simulink model "homing"  (R2017a)
settings: Solver=FixedStepAuto  StartTime=0.0  StopTime=inf  FixedStep=1e-3  RelTol=1e-3  EnableMultiTasking=on
libraries: xpcnilib x12, simulink x4
settings Model: SimulationMode=external  Creator=Davide  LastModifiedBy=stefa
settings SolverCC: EnableConcurrentExecution=on  ConcurrentTasks=on  AutoInsertRateTranBlk=on
settings DataIOCC: SaveFormat=StructureWithTime
settings OptimizationCC: BlockReduction=off  OptimizeBlockIOStorage=off  BufferReuse=off  GlobalBufferReuse=off  ExpressionFolding=off  LocalBlockOutputs=off
settings HardwareCC: ProdBitPerPointer=32  ProdBitPerSizeT=32  ProdBitPerPtrDiffT=32  ProdLargestAtomicFloat=None  ProdWordSize=32  ProdLongLongMode=on  ProdHWDeviceType=Generic->32-bit x86 compatible
settings RTWCC: SystemTargetFile=slrt.tlc  TemplateMakefile=slrt_default_tmf  Description=Simulink Real-Time  RTWCompilerOptimization=on
settings SimulinkRealTimeCC: xPCConcurrentTasks=on

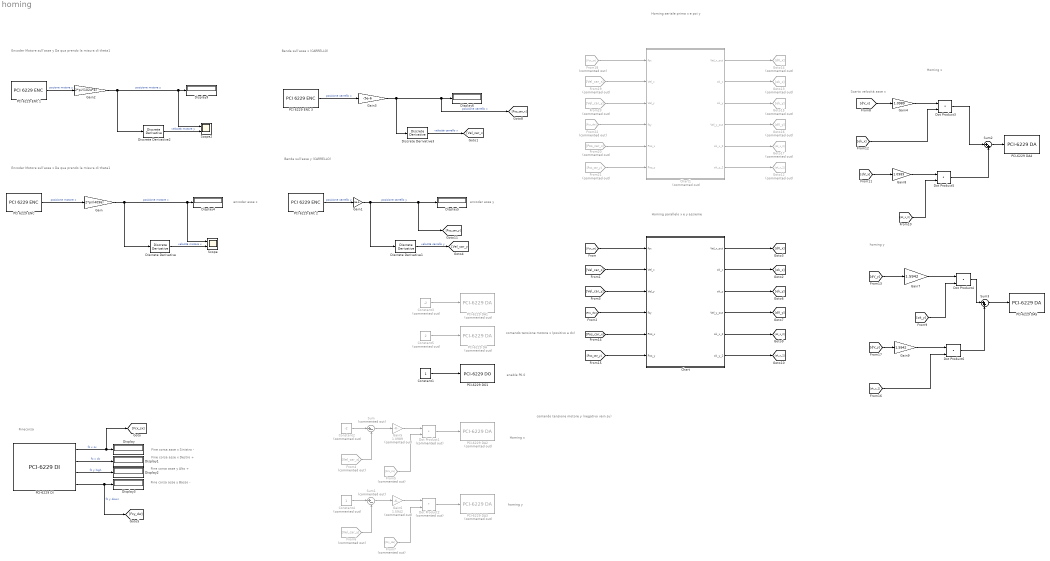
== system homing ==
  note: Homing seriale
      | prima x e poi y
  note: Scarto velocità asse x
  note: Encoder Motore sull'asse x
      | Da qua prendo la misura di theta1
  note: Fine corsa asse x Sinistro -
  note: homing y
  note: Homing x
  note: enable P0.0
  note: comando tensione motore x (positivo a dx)
  note: comando tensione motore y (negativo vain su)
  note: Finecorsa
  note: encoder asse y
  note: encoder asse x
  note: Fine corsa asse x Destro +
  note: Fine corsa asse y Alto +
  note: Fine corsa asse y Basso -
  note: Encoder Motore sull'asse y
      | Da qua prendo la misura di theta1
  note: Banda sull'asse x (CARRELLO)
  note: Banda sull'asse y (CARRELLO)
  note: Homing x
  note: homing y
  note: Homing parallelo
      | x e y assieme
  Chart : Stateflow chart  TreatAsAtomicUnit=on
  Chart1 : Stateflow chart  Commented=on  TreatAsAtomicUnit=on
  Constant1 : Constant
  Constant2 : Constant  Commented=on  Value=-2
  Constant3 : Constant  Commented=on  Value=-2
  Constant4 : Constant  Commented=on
  Constant5 : Constant  Commented=on  Value=2
  Discrete Derivative{,1..3} (4 alike) : simulink/Discrete/Discrete Derivative  gainval=1.0  ICPrevScaledInput=0.0  OutMin=[]  OutMax=[]  OutDataType=fixdt(1, 16)  OutScaling=2^-10  DoSatur=off
  Display{,1..6,9} (8 alike) : Display
  Dot Product1 : DotProduct  Commented=on  InputSameDT=on  OutDataTypeStr=Inherit: Inherit via internal rule
  Dot Product2 : DotProduct  Commented=on  InputSameDT=on  OutDataTypeStr=Inherit: Inherit via internal rule
  Dot Product{3..6} (4 alike) : DotProduct  InputSameDT=on  OutDataTypeStr=Inherit: Inherit via internal rule
  From18 : From  Commented=on  GotoTag=Fcx_sx
  From19 : From  Commented=on  GotoTag=Vel_car_x
  From20 : From  Commented=on  GotoTag=Pos_car_x
  From21 : From  Commented=on  GotoTag=Pos_car_y
  From22 : From  Commented=on  GotoTag=Fcy_dw
  From23 : From  Commented=on  GotoTag=Vel_car_y
  From4 : From  Commented=on  GotoTag=Vel_car_x
  From5 : From  Commented=on  GotoTag=Fcx_sx
  From6 : From  Commented=on  GotoTag=Vel_car_y
  From7 : From  Commented=on  GotoTag=Fcy_dw
  Gain : Gain  Gain=2*pi/(4096)
  Gain1 : Gain  Gain=-5e-6
  Gain2 : Gain  Gain=2*pi/(1024*4)
  Gain3 : Gain  Gain=-5e-6
  Gain4 : Gain  Gain=1.0989
  Gain5 : Gain  Commented=on  Gain=1.0989
  Gain6 : Gain  Commented=on  Gain=1.5942
  Gain7 : Gain  Gain=1.5942
  Gain8 : Gain  Gain=1.0989
  Gain9 : Gain  Gain=1.5942
  Goto12 : Goto  Commented=on  GotoTag=ok_y_2
  Goto13 : Goto  Commented=on  GotoTag=ok_x
  Goto14 : Goto  Commented=on  GotoTag=dV_x
  Goto15 : Goto  Commented=on  GotoTag=ok_y
  Goto16 : Goto  Commented=on  GotoTag=dV_y
  Goto17 : Goto  Commented=on  GotoTag=ok_x_2
  "PCI 6229 ENC " : xpcnilib/Incremental Encoder/PCI 6229 ENC   channel=0  countMode=Quadrature Mode x4  initCount=0  reload=on  indexPhase=A low B low  filter=None  sampleTime=0.001  slot=[4 12]
      settings: SourceProductName=Simulink Real-Time  SourceProductBaseCode=XP
  PCI 6229 ENC 1 : xpcnilib/Incremental Encoder/PCI 6229 ENC   channel=1  countMode=Quadrature Mode x4  initCount=0  reload=on  indexPhase=A low B low  filter=None  sampleTime=0.001  slot=[4 12]
      settings: SourceProductName=Simulink Real-Time  SourceProductBaseCode=XP
  PCI 6229 ENC 2 : xpcnilib/Incremental Encoder/PCI 6229 ENC   channel=0  countMode=Quadrature Mode x4  initCount=0  reload=on  indexPhase=A low B low  filter=None  sampleTime=0.001  slot=[4 15]
      settings: SourceProductName=Simulink Real-Time  SourceProductBaseCode=XP
  PCI 6229 ENC 3 : xpcnilib/Incremental Encoder/PCI 6229 ENC   channel=1  countMode=Quadrature Mode x4  initCount=0  reload=on  indexPhase=A low B low  filter=None  sampleTime=0.001  slot=[4 15]
      settings: SourceProductName=Simulink Real-Time  SourceProductBaseCode=XP
  PCI-6229 DA : xpcnilib/D//A/M Series/PCI-6229 DA  Commented=on  channel=[1]  reset=[1]  initValue=[0]  sampletime=0.001  slot=[4 12]
      settings: SourceProductName=Simulink Real-Time  SourceProductBaseCode=XP
  PCI-6229 DA1 : xpcnilib/D//A/M Series/PCI-6229 DA  Commented=on  channel=[1]  reset=[1]  initValue=[0]  sampletime=0.001  slot=[4 15]
      settings: SourceProductName=Simulink Real-Time  SourceProductBaseCode=XP
  PCI-6229 DA2 : xpcnilib/D//A/M Series/PCI-6229 DA  Commented=on  channel=[1]  reset=[1]  initValue=[0]  sampletime=0.001  slot=[4 12]
      settings: SourceProductName=Simulink Real-Time  SourceProductBaseCode=XP
  PCI-6229 DA3 : xpcnilib/D//A/M Series/PCI-6229 DA  Commented=on  channel=[1]  reset=[1]  initValue=[0]  sampletime=0.001  slot=[4 15]
      settings: SourceProductName=Simulink Real-Time  SourceProductBaseCode=XP
  PCI-6229 DA4 : xpcnilib/D//A/M Series/PCI-6229 DA  channel=[1]  reset=[1]  initValue=[0]  sampletime=0.001  slot=[4 12]
      settings: SourceProductName=Simulink Real-Time  SourceProductBaseCode=XP
  PCI-6229 DA5 : xpcnilib/D//A/M Series/PCI-6229 DA  channel=[1]  reset=[1]  initValue=[0]  sampletime=0.001  slot=[4 15]
      settings: SourceProductName=Simulink Real-Time  SourceProductBaseCode=XP
  PCI-6229 DI : xpcnilib/Digital Input/M Series/PCI-6229 DI  channel=[4 5 6 7]  sampletime=0.001  slot=[4 12]
      settings: SourceProductName=Simulink Real-Time  SourceProductBaseCode=XP
  PCI-6229 DO1 : xpcnilib/Digital Output/M Series/PCI-6229 DO  channel=[1]  reset=[1]  initValue=[0]  sampletime=0.001  slot=[4 12]
      settings: SourceProductName=Simulink Real-Time  SourceProductBaseCode=XP
  Scope : Scope  NumInputPorts=2
  Scope2 : Scope  NumInputPorts=2
  Sum : Sum  Commented=on  Inputs=|+-
  Sum1 : Sum  Commented=on  Inputs=|+-
  Sum2 : Sum  Inputs=|++
  Sum3 : Sum  Inputs=|++
  wires:
  PCI-6229 DI/1 -> [Fcx_sx], Display/1  "fc x sx"
  PCI-6229 DI/2 -> Display1/1  "fc x dx"
  PCI-6229 DI/3 -> Display2/1  "fc y high"
  PCI-6229 DI/4 -> [Fcy_dw], Display3/1  "fc y down"
  PCI 6229 ENC 1/1 -> Gain2/1  "pozione motore y"
  PCI 6229 ENC 3/1 -> Gain3/1  "posizione carrello x"
  PCI 6229 ENC 2/1 -> Gain1/1  "posizione carrello y"
  "PCI 6229 ENC "/1 -> Gain/1  "posizione motore x"
  Discrete Derivative/1 -> Scope/2  "velocità motore x"
  Discrete Derivative1/1 -> [Vel_car_y]  "velocità carrello y"
  Gain/1 -> Display4/1, Scope/1, Discrete Derivative/1  "posizione motore x"
  Gain1/1 -> [Pos_car_y], Display5/1, Discrete Derivative1/1  "posizione carrello y"
  Gain2/1 -> Scope2/1, Display9/1, Discrete Derivative2/1  "posizione motore y"
  Gain3/1 -> Discrete Derivative3/1, [Pos_car_x], Display6/1  "posizione carrello x"
  Constant1/1 -> PCI-6229 DO1/1
  Constant3/1 -> PCI-6229 DA1/1
  Discrete Derivative2/1 -> Scope2/2  "velocità motore y"
  Discrete Derivative3/1 -> [Vel_car_x]  "velocità carrello x"
  [Fcx_sx] -> Chart/1(fcx)
  [Vel_car_x] -> Chart/2(Vel_x)
  Chart/1(Vel_x_out) -> [dV_x]
  Constant2/1 -> Sum/1
  From4/1 -> Sum/2
  Sum/1 -> Gain5/1
  Gain5/1 -> Dot Product1/1
  Dot Product1/1 -> PCI-6229 DA2/1
  From5/1 -> Dot Product1/2
  Constant4/1 -> Sum1/1
  Gain6/1 -> Dot Product2/1
  Sum1/1 -> Gain6/1
  Dot Product2/1 -> PCI-6229 DA3/1
  From6/1 -> Sum1/2
  From7/1 -> Dot Product2/2
  Constant5/1 -> PCI-6229 DA/1
  [Fcy_dw] -> Chart/4(fcy)
  [Vel_car_y] -> Chart/3(Vel_y)
  Chart/2(ok_x) -> [ok_x]
  Chart/3(ok_y) -> [ok_y]
  Chart/4(Vel_y_out) -> [dV_y]
  [dV_y] -> Gain7/1
  Gain4/1 -> Dot Product3/1
  [ok_x] -> Dot Product3/2
  [ok_y] -> Dot Product4/2
  Gain7/1 -> Dot Product4/1
  [dV_x] -> Gain4/1
  Dot Product5/1 -> Sum2/2
  [ok_x_2] -> Dot Product5/2
  Gain8/1 -> Dot Product5/1
  [dV_x] -> Gain8/1
  [Pos_car_x] -> Chart/5(Pos_x)
  Chart/5(ok_x_2) -> [ok_x_2]
  Sum2/1 -> PCI-6229 DA4/1
  Dot Product3/1 -> Sum2/1
  Chart/6(ok_y_2) -> [ok_y_2]
  [Pos_car_y] -> Chart/6(Pos_y)
  [dV_y] -> Gain9/1
  Gain9/1 -> Dot Product6/1
  [ok_y_2] -> Dot Product6/2
  Dot Product6/1 -> Sum3/2
  Sum3/1 -> PCI-6229 DA5/1
  Dot Product4/1 -> Sum3/1
  From21/1 -> Chart1/6(Pos_y)
  Chart1/6(ok_y_2) -> Goto12/1
  From22/1 -> Chart1/4(fcy)
  Chart1/2(ok_x) -> Goto13/1
  From19/1 -> Chart1/2(Vel_x)
  From20/1 -> Chart1/5(Pos_x)
  From23/1 -> Chart1/3(Vel_y)
  Chart1/3(ok_y) -> Goto15/1
  Chart1/1(Vel_x_out) -> Goto14/1
  From18/1 -> Chart1/1(fcx)
  Chart1/4(Vel_y_out) -> Goto16/1
  Chart1/5(ok_x_2) -> Goto17/1

== stateflow chart homing/Chart1 ==
  state Homing
    state Homing_x
      entry:
      v_sp_x=-2.1;
      ok_x=1;
      ok_x_2=0;
      during:
      Vel_x_out = v_sp_x-Vel_x;
    note: Inizializzazione asse x
        | asse x -> 0
        |
        | Vel_x = velocità carrello
        | ok_x = abilito motore torna indietro
        | ok_x_2 = disaabilito motore va in avant
        | Vel_x_out = scarto velocità x
    note: Passo sull'asse y solo quando il fine corsa sinistro è attivo
    state Homing_y
      entry:
      ok_x=0;
      v_sp_y=1.2;
      ok_y=1;
      during:
      Vel_y_out=v_sp_y-Vel_y;
    note: Inizializzazione asse y
        | asse y -> 0
        | ok_x = disabilito motore asse x indietro
        | ok_y = abilito motorey va sopra
        | Vel_y_out = scarto velocità y
    note: Fine inizializzazione
    state Fine_homing1
      entry:
      ok_y=0;
      ok_x=0;
      bx=Pos_x;
      v_sp_x=2.1;
      ok_x_2=1;
      during:
      Vel_x_out=v_sp_x-Vel_x;
      dx=Pos_x-bx
    note: Porto al centro asse x
        | asse y (fermo)
        | ok_x = disabilito motore asse x indietro
        | ok_y = disabilito motorey va sopra
        | bx = posizione carrello assex iniziale
        | ok_x_2 = abilitato motore avanti
        | Vel_x_out = scarto velocità
        | dx= calcolo distanza da pos. iniziale
    state Posizionamento_y
      entry:
      ok_x_2=0;
      by=Pos_y;
      v_sp_y=-1.2;
      ok_y_2=1;
      during:
      Vel_y_out=v_sp_y-Vel_y;
      dy=abs(Pos_y-by);
    note: Porto al centro asse y
        | asse x (fermo)
        | ok_x = disabilito motore asse x indietro
        | ok_y = disabilito motorey va sopra
        | by = posizione carrello assex iniziale
        | ok_x_2 = abilitato motore avanti
        | Vel_x_out = scarto velocità
        | dx= calcolo distanza da pos. iniziale
    state Fine
      entry:
      ok_y_2=0;
      ok_x_2=0;
    (default) -> Homing_x
    Homing_x -> Homing_y : [fcx==0]
    Homing_y -> Fine_homing1 : [fcy==0]
    Fine_homing1 -> Posizionamento_y : [dx>0.5]
    Posizionamento_y -> Fine : [dy>0.5]
  (default) -> Homing
  data: fcx input; Vel_x_out output; Vel_x input; ok_x output; ok_y output; Vel_y input; Vel_y_out output; fcy input; Pos_x input; dx local; ok_x_2 output; v_sp_x local; v_sp_y local; Pos_y input; ok_y_2 output; dy local; bx local; by local

== stateflow chart homing/Chart ==
  state Homing
    state Homing_x
      entry:
      v_sp_x=-2.1;
      v_sp_y=1.2;
      ok_x=1;
      ok_y=1;
      ok_x_2=0;
      during:
      Vel_x_out = v_sp_x-Vel_x;
      Vel_y_out=v_sp_y-Vel_y;
    note: Inizializzazione asse x
        | asse x -> 0
        |
        | Vel_x = velocità carrello
        | ok_x = abilito motore torna indietro
        | ok_x_2 = disaabilito motore va in avant
        | Vel_x_out = scarto velocità x
    note: Passo sull'asse y solo quando il fine corsa sinistro è attivo
    note: Inizializzazione asse y
        | asse y -> 0
        | ok_x = disabilito motore asse x indietro
        | ok_y = abilito motorey va sopra
        | Vel_y_out = scarto velocità y
    note: Fine inizializzazione
    state Fine_homing1
      entry:
      ok_y=0;
      ok_x=0;
      bx=Pos_x;
      by=Pos_y;
      v_sp_x=2.1;
      v_sp_y=-1.2;
      ok_x_2=1;
      ok_y_2=1;
      during:
      Vel_x_out=v_sp_x-Vel_x;
      dx=Pos_x-bx
      if (dx>0.5 )
      Vel_x_out=0;
      end
      Vel_y_out=v_sp_y-Vel_y;
      dy=abs(Pos_y-by);
      if (dy>0.5 )
      Vel_y_out=0;
      end
    note: Porto al centro asse x
        | asse y (fermo)
        | ok_x = disabilito motore asse x indietro
        | ok_y = disabilito motorey va sopra
        | bx = posizione carrello assex iniziale
        | ok_x_2 = abilitato motore avanti
        | Vel_x_out = scarto velocità
        | dx= calcolo distanza da pos. iniziale
    note: Porto al centro asse y
        | asse x (fermo)
        | ok_x = disabilito motore asse x indietro
        | ok_y = disabilito motorey va sopra
        | by = posizione carrello assex iniziale
        | ok_x_2 = abilitato motore avanti
        | Vel_x_out = scarto velocità
        | dx= calcolo distanza da pos. iniziale
    state Fine
      entry:
      ok_y_2=0;
      ok_x_2=0;
    (default) -> Homing_x
    Homing_x -> Fine_homing1 : [fcx==0 && fcy==0]
    Fine_homing1 -> Fine : [dx>0.5 && dy>0.5]
  (default) -> Homing
  data: fcx input; Vel_x_out output; Vel_x input; ok_x output; ok_y output; Vel_y input; Vel_y_out output; fcy input; Pos_x input; dx local; ok_x_2 output; v_sp_x local; v_sp_y local; Pos_y input; ok_y_2 output; dy local; bx local; by local
